simulink model "FFR_1_1"  (R2015a)
settings: Solver=ode45  StartTime=0.0  StopTime=15  RelTol=1e-3
values from neighbouring files (symbols this model uses):
  D = 0.015    [init_FFR_1_0.m]    (also in init_FFR_1_1.m; init_FFR_3area.m = [0.015 0.016 0.015]; init_FFR_3area_2.m = [0.015 0.016 0.015]; init_FFR_3area_3.m = [0.015 0.016 0.015])
  D_filter = 100    [init_FFR_1_1.m]
  H = 0.0833    [init_FFR_1_0.m]    (also in init_FFR_1_1.m; init_FFR_3area.m = [0.1667 0.2017 0.1247] .* 0.5; init_FFR_3area_2.m = [0.1667 0.2017 0.1247] .* 0.5; init_FFR_3area_3.m = [0.1667 0.2017 0.1247] .* 0.5)
  Kd = -1    [init_FFR_1_1.m]
  Ki = -0.3    [init_FFR_1_0.m]    (also in init_FFR_1_1.m = -2; init_FFR_3area.m = [-0.3 -0.2 -0.4]; init_FFR_3area_2.m = [-0.3 -0.2 -0.4]; init_FFR_3area_3.m = [-0.3 -0.2 -0.4])
  Kp = -0.5    [init_FFR_1_1.m]    (also in init_FRR_3area_6.m = [-0.5 -0.5 -0.5]; init_FRR_4area_1.m = [0 0 0 0])
  R = 3    [init_FFR_1_0.m]    (also in init_FFR_1_1.m; init_FFR_3area.m = [3 2.73 2.82]; init_FFR_3area_2.m = [3 2.73 2.82]; init_FFR_3area_3.m = [3 2.73 2.82])
  T_g = 0.08    [init_FFR_1_0.m]    (also in init_FFR_1_1.m; init_FFR_3area.m = [0.08 0.06 0.07]; init_FFR_3area_2.m = [0.08 0.06 0.07]; init_FFR_3area_3.m = [0.08 0.06 0.07])
  T_t = 0.40    (= 0.4)    [init_FFR_1_0.m]    (also in init_FFR_1_1.m; init_FFR_3area.m = [0.40 0.44 0.30]; init_FFR_3area_2.m = [0.40 0.44 0.30]; init_FFR_3area_3.m = [0.40 0.44 0.30])
libraries: simulink x1
settings Model: Creator=tarje  LastModifiedBy=tarje

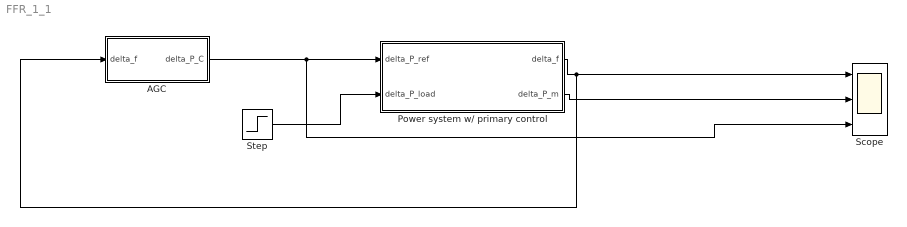
== system FFR_1_1 ==
  AGC : Subsystem
  Power system w/ primary control : Subsystem
  Scope : Scope  NumInputPorts=3
      settings: TimeRange=15  YMin=-0.08~-0.005~-0.01  YMax=0.025~0.04~0.03
  Step : Step  Time=2  After=0.02  SampleTime=0
  wires:
  Step/1 -> Power system w/ primary control/2(delta_P_load)
  Power system w/ primary control/1(delta_f) -> AGC/1(delta_f), Scope/1
  Power system w/ primary control/2(delta_P_m) -> Scope/2
  AGC/1(delta_P_C) -> Scope/3, Power system w/ primary control/1(delta_P_ref)

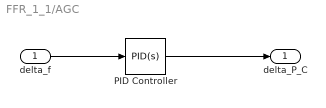
== system FFR_1_1/AGC ==
  delta_f : Inport
  PID Controller : simulink/Continuous/PID Controller  Controller=PID  TimeDomain=Continuous-time  SampleTime=-1  IntegratorMethod=Forward Euler  FilterMethod=Forward Euler  Form=Parallel  UseFilter=on  ControllerParametersSource=internal  P=Kp  I=Ki  D=Kd  N=D_filter  InitialConditionSource=internal  InitialConditionForIntegrator=0  InitialConditionForFilter=0  ExternalReset=none  LimitOutput=off  UpperSaturationLimit=inf  LowerSaturationLimit=-inf  LinearizeAsGain=on  AntiWindupMode=none  Kb=1  TrackingMode=off  Kt=1  PParamMin=[]  PParamMax=[]  IParamMin=[]  IParamMax=[]  DParamMin=[]  DParamMax=[]  NParamMin=[]  NParamMax=[]  KbParamMin=[]  KbParamMax=[]  KtParamMin=[]  KtParamMax=[]  POutMin=[]  POutMax=[]  IOutMin=[]  IOutMax=[]  DOutMin=[]  DOutMax=[]  NOutMin=[]  NOutMax=[]  KbOutMin=[]  KbOutMax=[]  KtOutMin=[]  KtOutMax=[]  IntegratorOutMin=[]  IntegratorOutMax=[]  FilterOutMin=[]  FilterOutMax=[]  SumOutMin=[]  SumOutMax=[]  SumI1OutMin=[]  SumI1OutMax=[]  SumI2OutMin=[]  SumI2OutMax=[]  SumI3OutMin=[]  SumI3OutMax=[]  SumDOutMin=[]  SumDOutMax=[]  SaturationOutMin=[]  SaturationOutMax=[]  IntegratorContinuousStateAttributes=''  IntegratorStateMustResolveToSignalObject=off  IntegratorRTWStateStorageClass=Auto  FilterContinuousStateAttributes=''  FilterStateMustResolveToSignalObject=off  FilterRTWStateStorageClass=Auto  DifferentiatorICPrevScaledInput=0  DifferentiatorOutMin=[]  DifferentiatorOutMax=[]
  delta_P_C : Outport
  wires:
  delta_f/1 -> PID Controller/1
  PID Controller/1 -> delta_P_C/1

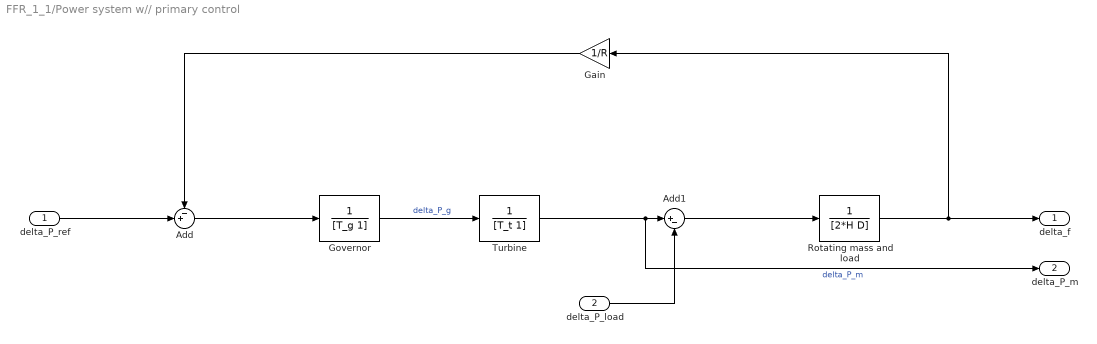
== system FFR_1_1/Power system w// primary control ==
  delta_P_ref : Inport
  delta_P_load : Inport  Port=2
  Add : Sum  Inputs=-+|
  Add1 : Sum  Inputs=|+-
  Gain : Gain  Gain=1/R
  Governor : TransferFcn  Denominator=[T_g 1]
  Rotating mass and load : TransferFcn  Denominator=[2*H D]
  Turbine : TransferFcn  Denominator=[T_t 1]
  delta_f : Outport
  delta_P_m : Outport  Port=2
  wires:
  Turbine/1 -> delta_P_m/1, Add1/1  "delta_P_m"
  Rotating mass and load/1 -> delta_f/1, Gain/1
  Gain/1 -> Add/1
  delta_P_load/1 -> Add1/2
  Add1/1 -> Rotating mass and load/1
  Add/1 -> Governor/1
  Governor/1 -> Turbine/1  "delta_P_g"
  delta_P_ref/1 -> Add/2
